simulink model "MCuC_CAN_codegen"  (R2023b)
settings: Solver=FixedStepAuto  StartTime=0.0  StopTime=10.0  RelTol=1e-3
settings Model: Creator=rebek  LastModifiedBy=rebek
settings OptimizationCC: DefaultParameterBehavior=Inlined  EnhancedBackFolding=on  PassReuseOutputArgsAs=Individual arguments  ZeroExternalMemoryAtStartup=off  ZeroInternalMemoryAtStartup=off  OptimizeBlockOrder=speed  DifferentSizesBufferReuse=on  OptimizationCustomize=off  EfficientTunableParamExpr=on
settings DebuggingCC: ParameterTunabilityLossMsg=error
settings SFSimCC: MATLABDynamicMemAlloc=off
settings RTWCC: Description=Embedded Coder  SystemTargetFile=ert.tlc  GenCodeOnly=on  TemplateMakefile=ert_default_tmf  TargetLang=C++
settings CodeAppCC: ForceParamTrailComments=on  IgnoreCustomStorageClasses=off  OperatorAnnotations=on  SimulinkDataObjDesc=on  SFDataObjDesc=on  InsertBlockDesc=on
settings ERTTargetCC: TargetLangStandard=C++11 (ISO)  GenerateSampleERTMain=on  CodeInterfacePackaging=C++ class  InlinedParameterPlacement=NonHierarchical  RootIOFormat=Structure reference  ERTCustomFileTemplate=example_file_process.tlc

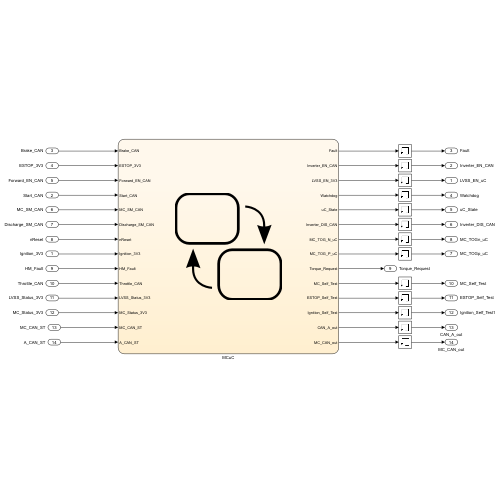
[thumbnail: Simulink's stored preview of the top-level diagram]
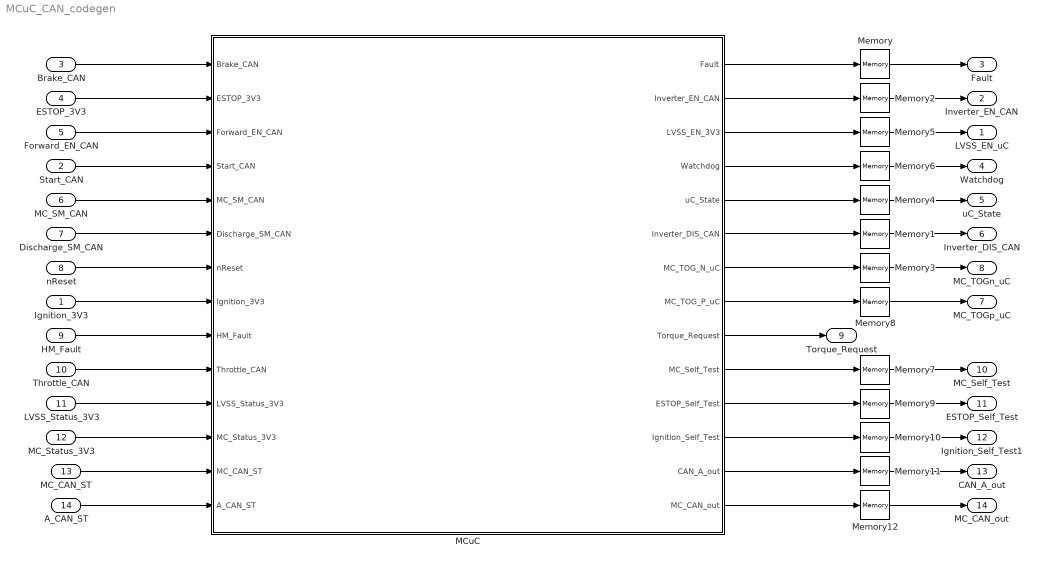
== system MCuC_CAN_codegen ==
  Ignition_3V3 : Inport  OutDataTypeStr=boolean
  Start_CAN : Inport  Port=2  OutDataTypeStr=boolean
  Brake_CAN : Inport  Port=3  OutDataTypeStr=boolean
  ESTOP_3V3 : Inport  Port=4  OutDataTypeStr=boolean
  Forward_EN_CAN : Inport  Port=5  OutDataTypeStr=boolean
  MC_SM_CAN : Inport  Port=6  OutDataTypeStr=uint8
  Discharge_SM_CAN : Inport  Port=7  OutDataTypeStr=uint8
  nReset : Inport  Port=8  OutDataTypeStr=boolean
  HM_Fault : Inport  Port=9  OutDataTypeStr=boolean
  Throttle_CAN : Inport  Port=10  OutDataTypeStr=uint16
  LVSS_Status_3V3 : Inport  Port=11  OutDataTypeStr=boolean
  MC_Status_3V3 : Inport  Port=12  OutDataTypeStr=boolean
  MC_CAN_ST : Inport  Port=13  OutDataTypeStr=boolean
  A_CAN_ST : Inport  Port=14  OutDataTypeStr=boolean
  MCuC : Stateflow chart  TreatAsAtomicUnit=on
      settings: PortSchema="{\"entries\":[{\"content\":{\"sides\":[{\"content\":{\"connectorIds\":[\"In1\",\"In2\",\"In3\",\"In5\",\"In6\",\"In7\",\"In8\",\"In4\",\"In9\",\"In10\",\"In11\",\"In12\",\"In13\",\"In14\"]},\"type\":\"ConnectorPlacement.EquallySpacedRectSide\",\"uuid\":\"d1510c73-f1c7-4e03-bb6c-bda7856f993e\"},{\"content\":{\"connectorIds\":[\"Out1\",\"Out2\",\"Out3\",\"Out4\",\"Out5\",\"Out6\",\"Out7\",\"Out8\",\"Out9\",\"Out10\",\"Out11\",\"Out12\",\"Out13\",\"Out14\"],\"side\":\"RIGHT\"},\"type\":\"ConnectorPlacement.EquallySpacedRectSide\",\"uuid\":\"1a7878c4-a817-4ca0-b21c-0429e82bb9d7\"},{\"content\":{\"side\":\"TOP\"},\"type\":\"ConnectorPlacement.EquallySpacedRectSide\",\"uuid\":\"ed9f2701-7044-4bb4-9c0b-b9cf9840e69e\"}]},\"type\":\"ConnectorPlacement.EquallySpacedConnector\",\"uuid\":\"4ceb8e7d-629c-4438-88a9-aa3016537644\"}],\"packageUris\":[\"http://schema.mathworks.com/mf0/Connector/R2020b\"],\"version\":\"1.0\"}"
  Memory{,1..12} (13 alike) : Memory
  LVSS_EN_uC : Outport  OutDataTypeStr=boolean
  Inverter_EN_CAN : Outport  Port=2  OutDataTypeStr=boolean
  Fault : Outport  Port=3  OutDataTypeStr=boolean
  Watchdog : Outport  Port=4  OutDataTypeStr=boolean
  uC_State : Outport  Port=5  OutDataTypeStr=uint8
  Inverter_DIS_CAN : Outport  Port=6  OutDataTypeStr=boolean
  MC_TOGp_uC : Outport  Port=7  OutDataTypeStr=boolean
  MC_TOGn_uC : Outport  Port=8  OutDataTypeStr=boolean
  Torque_Request : Outport  Port=9  OutDataTypeStr=uint16
  MC_Self_Test : Outport  Port=10  OutDataTypeStr=boolean
  ESTOP_Self_Test : Outport  Port=11  OutDataTypeStr=boolean
  Ignition_Self_Test1 : Outport  Port=12  OutDataTypeStr=boolean
  CAN_A_out : Outport  Port=13  OutDataTypeStr=boolean
  MC_CAN_out : Outport  Port=14  OutDataTypeStr=boolean
  wires:
  MCuC/12(Ignition_Self_Test) -> Memory10/1
  MCuC/14(MC_CAN_out) -> Memory12/1
  Start_CAN/1 -> MCuC/5(Start_CAN)
  MCuC/7(MC_TOG_N_uC) -> Memory3/1
  Memory12/1 -> MC_CAN_out/1
  Memory8/1 -> MC_TOGp_uC/1
  Memory9/1 -> ESTOP_Self_Test/1
  MCuC/8(MC_TOG_P_uC) -> Memory8/1
  nReset/1 -> MCuC/8(nReset)
  Forward_EN_CAN/1 -> MCuC/3(Forward_EN_CAN)
  MCuC/6(Inverter_DIS_CAN) -> Memory1/1
  MC_Status_3V3/1 -> MCuC/12(MC_Status_3V3)
  MCuC/2(Inverter_EN_CAN) -> Memory2/1
  MCuC/1(Fault) -> Memory/1
  Memory6/1 -> Watchdog/1
  MCuC/3(LVSS_EN_3V3) -> Memory5/1
  MCuC/5(uC_State) -> Memory4/1
  Memory/1 -> Fault/1
  MCuC/4(Watchdog) -> Memory6/1
  Memory7/1 -> MC_Self_Test/1
  Memory1/1 -> Inverter_DIS_CAN/1
  LVSS_Status_3V3/1 -> MCuC/11(LVSS_Status_3V3)
  Memory3/1 -> MC_TOGn_uC/1
  Memory5/1 -> LVSS_EN_uC/1
  Memory4/1 -> uC_State/1
  HM_Fault/1 -> MCuC/9(HM_Fault)
  MC_CAN_ST/1 -> MCuC/13(MC_CAN_ST)
  MCuC/11(ESTOP_Self_Test) -> Memory9/1
  Brake_CAN/1 -> MCuC/1(Brake_CAN)
  MCuC/9(Torque_Request) -> Torque_Request/1
  A_CAN_ST/1 -> MCuC/14(A_CAN_ST)
  Memory11/1 -> CAN_A_out/1
  Memory10/1 -> Ignition_Self_Test1/1
  Discharge_SM_CAN/1 -> MCuC/7(Discharge_SM_CAN)
  Memory2/1 -> Inverter_EN_CAN/1
  MCuC/13(CAN_A_out) -> Memory11/1
  MC_SM_CAN/1 -> MCuC/6(MC_SM_CAN)
  MCuC/10(MC_Self_Test) -> Memory7/1
  Throttle_CAN/1 -> MCuC/10(Throttle_CAN)
  ESTOP_3V3/1 -> MCuC/2(ESTOP_3V3)
  Ignition_3V3/1 -> MCuC/4(Ignition_3V3)

== stateflow chart MCuC_CAN_codegen/MCuC ==
  state MCuC
    state MCuC_Logic [parallel]
      settings: executionOrder=1
      state ESTOP
        entry:
        uC_State = 7;
        LVSS_EN_3V3 = false;
        ESTOP_activated = false;
      state MC_Off
        entry:
        LVSS_EN_3V3 = false;
        uC_State = 0;
        uncharged = true;
        Inverter_EN_CAN = false;
        MC_Self_Test = false;
      state LVSS_MC_Shutdown
        entry:
        uC_State = 9;
        LVSS_EN_3V3 = false;
        Inverter_DIS_CAN = false;
        MC_TOG_P_uC = false;
        MC_TOG_N_uC = true;
        exit:
        MC_TOG_P_uC = false;
        MC_TOG_N_uC = false;
      state MC_Discharging
        entry:
        uC_State = 5;
      state Fault_Ignit_H
      state Fault
        entry:
        uC_State = 6;
        Fault_Activated = false;
        Fault = true;
        exit:
        Fault = false;
      state LVSS_MC_Startup
        entry:
        uncharged = false;
        uC_State = 8;
        LVSS_EN_3V3 = true;
        MC_TOG_P_uC = true;
        MC_TOG_N_uC = false;
        exit:
        MC_TOG_P_uC = false;
        MC_TOG_N_uC = false;
      state Setup
        entry:
        uC_State = 10;
        MC_Self_Test = true;
        state MC_ST
          state MC_ON
            entry:
            MC_TOG_P_uC = true;
            MC_TOG_N_uC = false;
          state MC_OFF
            entry:
            MC_TOG_P_uC = false;
            MC_TOG_N_uC = true;
          state MC_Fails
            entry:
            uC_State = 15;
            MC_TOG_P_uC = false;
            MC_TOG_N_uC = false;
          (default) -> MC_ON
          MC_ON -> MC_OFF [order 1] : [MC_Status_3V3 == true]
          MC_ON -> MC_Fails [order 2] : [MC_Status_3V3 == false && after(2,sec)]
          MC_OFF -> MC_Fails [order 1] : [MC_Status_3V3 == true && after(2,sec)]
        state Ignition_ST
          state Ignition_Low
            entry:
            Ignition_Self_Test = true;
          state Ignition_High
            entry:
            Ignition_Self_Test = false;
          state Ignition_Fails
            entry:
            uC_State = 14;
          (default) -> Ignition_Low
          Ignition_Low -> Ignition_High [order 1] : [Ignition_3V3 == false]
          Ignition_Low -> Ignition_Fails [order 2] : [Ignition_3V3 == true]
          Ignition_High -> Ignition_Fails [order 1] : [Ignition_3V3 == false]
        state ESTOP_ST
          state ESTOP_Low
            entry:
            ESTOP_Self_Test = true;
          state ESTOP_High
            entry:
            ESTOP_Self_Test = false;
          state ESTOP_Fails
            entry:
            uC_State = 13;
          (default) -> ESTOP_Low
          ESTOP_Low -> ESTOP_High [order 1] : [ESTOP_3V3 == false]
          ESTOP_Low -> ESTOP_Fails [order 2] : [ESTOP_3V3 == true]
          ESTOP_High -> ESTOP_Fails [order 1] : [ESTOP_3V3 == false]
        state MC_CAN_ST
          state MC_Transmit
            entry:
            MC_CAN_out = true;
          state MC_CAN_fails
            entry:
            uC_State = 12;
          (default) -> MC_Transmit
          MC_Transmit -> MC_CAN_fails [order 1] : [MC_CAN_ST == false && after(30,sec)]
        state CAN_A_ST
          state A_Transmit
            entry:
            CAN_A_out = true;
          state A_CAN_fails
            entry:
            uC_State = 11;
          (default) -> A_Transmit
          A_Transmit -> A_CAN_fails [order 2] : [A_CAN_ST ==false && after(30,sec)]
        (default) -> MC_ST
        MC_OFF -> Ignition_ST [order 2] : [MC_Status_3V3 == false]
        Ignition_High -> ESTOP_ST [order 2] : [Ignition_3V3 == true]
        ESTOP_High -> MC_CAN_ST [order 2] : [ESTOP_3V3 == true]
        MC_Transmit -> CAN_A_ST [order 2] : [MC_CAN_ST == true]
      state Contactor_Open
        entry:
        Inverter_EN_CAN = false;
        Inverter_DIS_CAN = true;
        uC_State = 4;
      state MC_Init
        entry:
        uC_State = 1;
      state MC_Active
        entry:
        Inverter_EN_CAN = true;
        uC_State = 3;
        Torque_Request = 0;
        during:
        Torque_Request = Throttle_CAN;
        exit:
        Torque_Request = 0;
      state Contactor_Closed
        entry:
        uC_State = 2;
        Inverter_EN_CAN = false;
      ESTOP -> MC_Off : [ESTOP_3V3 == true]
      LVSS_MC_Shutdown -> MC_Off : [MC_Status_3V3 == false && LVSS_Status_3V3 == false]
      MCuC_Logic -> ESTOP [order 3] : [ESTOP_3V3 == false && uncharged == true && nReset == true && uC_State ~= 10]
      Fault_Ignit_H -> MC_Off : [Ignition_3V3 == true]
      MC_Discharging -> LVSS_MC_Shutdown : [Discharge_SM_CAN == 4]
      A_Transmit -> MC_Off [order 1] : [A_CAN_ST == true && MC_Status_3V3 == false && Ignition_3V3 == true && LVSS_Status_3V3 == false]
      MC_Off -> LVSS_MC_Startup : [Ignition_3V3 == false]
      Contactor_Open -> MC_Discharging : [Discharge_SM_CAN ~= 0]
      Fault -> Fault_Ignit_H : [MC_Status_3V3 == false && Ignition_3V3 == false]
      MCuC_Logic -> Fault [order 4] : [HM_Fault == 1 && uncharged == 1 && uC_State ~= 10 && nReset == 1]
      (default) -> Setup
      LVSS_MC_Startup -> MC_Init : [MC_Status_3V3 == true && LVSS_Status_3V3 == true]
      MCuC_Logic -> Contactor_Open [order 1] : [HM_Fault == true && Ignition_3V3 == false && uncharged == false && Fault_Activated == false]{Fault_Activated = true}
      MCuC_Logic -> Contactor_Open [order 2] : [ESTOP_3V3 == false && uncharged == false && ESTOP_activated == false]{ESTOP_activated = true}
      MCuC_Logic -> Setup [order 5] : [nReset == false]
      MC_Init -> Contactor_Open [order 1] : [Ignition_3V3 == true]
      Contactor_Closed -> Contactor_Open [order 2] : [Ignition_3V3 == true]
      MC_Active -> Contactor_Open [order 2] : [Ignition_3V3 == true]
      MC_Init -> Contactor_Closed [order 2] : [MC_SM_CAN == 5]
      Contactor_Closed -> MC_Active [order 1] : [Start_CAN == true && Forward_EN_CAN == true && Brake_CAN == true && Throttle_CAN == false]
      MC_Active -> Contactor_Closed [order 1] : [Forward_EN_CAN == false]
    state Watchdog [parallel]
      settings: executionOrder=2
      state WD0
        entry:
        Watchdog = false;
      state WD1
        entry:
        Watchdog = true;
      (default) -> WD0
      WD0 -> WD1 : after(.5, sec)
      WD1 -> WD0 : after(.5, sec)
  data: Fault output boolean =0; Brake_CAN input boolean; ESTOP_3V3 input boolean; Forward_EN_CAN input boolean; Ignition_3V3 input boolean; Start_CAN input boolean; MC_SM_CAN input uint8; Inverter_EN_CAN output boolean =0; LVSS_EN_3V3 output boolean =0; Discharge_SM_CAN input uint8; nReset input boolean; Watchdog output boolean =0; uC_State output uint8 =0; uncharged local boolean =1; ESTOP_activated local boolean =0; HM_Fault input boolean; Throttle_CAN input uint16; Inverter_DIS_CAN output boolean =0; MC_TOG_N_uC output boolean =0; MC_TOG_P_uC output boolean =0; LVSS_Status_3V3 input boolean; MC_Status_3V3 input boolean; Torque_Request output uint16 =0; Fault_Activated local boolean =0; MC_Self_Test output boolean; ESTOP_Self_Test output boolean; Ignition_Self_Test output boolean; CAN_A_out output boolean; MC_CAN_out output boolean; MC_CAN_ST input boolean; A_CAN_ST input boolean
